simulink model "ITSC2021_CoupledPathFollowingSim_discrete"  (R2019b)
settings: Solver=FixedStepAuto  StartTime=0.0  StopTime=50  FixedStep=0.01  RelTol=1e-4  EnableMultiTasking=on
values from neighbouring files (symbols this model uses):
  friction_grid_cluster = [frictionGrid_Cluster_table.position_x, frictionGrid_Cluster_table.position_y, frictionGrid_Cluster_table.position_z, frictionGrid_Cluster_table.friction_coefficient]    [ITSC2021_runCoupledPathFollowingSim.m]
  inputTrajectory = inputTrajectory(unique_station_indices,:)    [ITSC2021_runCoupledPathFollowingSim.m]
  road_geometry = [sectionRef_table.east, sectionRef_table.north, sectionRef_table.up, sectionRef_table.grade, sectionRef_table.bank, road_geometry_radius, sectionRef_table.yaw]    [ITSC2021_runCoupledPathFollowingSim.m]
undefined symbols (not defined in the file or in its folder): DiscIntNeverNeededParam, flag, initial, mdlparam, mdlParam
libraries: simulink x6, autolibshared x1
(part 1 of 3)
settings Model: Creator=cbeal  LastModifiedBy=LimingGao
settings SolverCC: ZeroCrossAlgorithm=Adaptive
settings DataIOCC: SaveFormat=Array  SaveState=on  SaveTime=off  ReturnWorkspaceOutputs=off
settings OptimizationCC: ExpressionDepthLimit=2147483647  LifeSpan=inf
settings DebuggingCC: ReadBeforeWriteMsg=DisableAll  WriteAfterWriteMsg=DisableAll  WriteAfterReadMsg=DisableAll  UnderspecifiedInitializationDetection=Classic  MergeDetectMultiDrivingBlocksExec=none  SolverPrmCheckMsg=warning  MultiTaskDSMMsg=none  FcnCallInpInsideContextMsg=warning  StateNameClashWarn=warning  SFUnexpectedBacktrackingDiag=warning  SFNoUnconditionalDefaultTransitionDiag=warning  SFExecutionAtInitializationDiag=none  ArithmeticOperatorsInVariantConditions=warning
settings HardwareCC: ProdBitPerPointer=32  ProdBitPerSizeT=32  ProdBitPerPtrDiffT=32  ProdLargestAtomicFloat=None  ProdIntDivRoundTo=Undefined  ProdEndianess=Unspecified  ProdWordSize=32  ProdHWDeviceType=32-bit Generic
settings ModelReferenceCC: UpdateModelReferenceTargets=IfOutOfDate  PropagateSignalLabelsOutOfModel=off
settings SFSimCC: SFSimEcho=off  SimUseLocalCustomCode=off  CustomCodeUndefinedFunction=UseInterfaceOnly
settings RTWCC: RTWUseLocalCustomCode=off
settings CodeAppCC: StateflowObjectComments=on
settings GRTTargetCC: TargetLangStandard=C89/C90 (ANSI)  GeneratePreprocessorConditionals=Disable all
settings ConfigComp: CovMetricSettings=dw  CovHtmlReporting=on  CovSaveCumulativeToWorkspaceVar=on  CovSaveSingleToWorkspaceVar=on  CovExternalEMLEnable=off

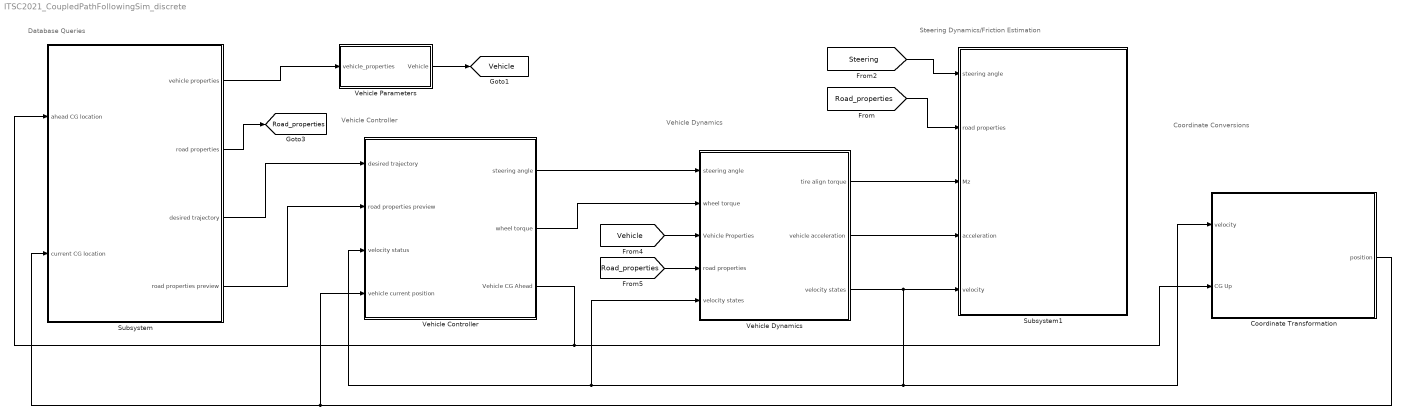
== system ITSC2021_CoupledPathFollowingSim_discrete ==
  note: Steering Dynamics/Friction Estimation
  note: Database Queries
  note: Vehicle Dynamics
  note: Vehicle Controller
  note: Coordinate Conversions
  Coordinate Transformation : Subsystem
  Subsystem : Subsystem
  Subsystem1 : Subsystem
  Vehicle Controller : Subsystem
      mask Display: image('Simulink_MaskIcons\driving_model_icon.png'); % Use "Edit Image" on toolstrip to change.
  Vehicle Dynamics : Subsystem
      mask Display: image('Simulink_MaskIcons\Vehicle_Newton_icon.png'); % Use "Edit Image" on toolstrip to change.
  Vehicle Parameters : Subsystem  mask{vehicleName='C5 Vette', m=1600, m_s=1600, Ixx=0, Iyy=0, Izz=2500, Iw=1.2, Re=0.32, a=1.3, b=1.3, d=1.5, h_cg=0.42, h_rcf=0, h_rcr=0, k_phi=0, b_phi=0, Ca=[95000; 95000; 110000; 110000], Cx=[65000,65000,65000,65000], mu_peak=[1.2 1.2 1.2 1.2], mu_slide=[0.9 0.9 0.9 0.9]}
      mask prompts: vehicleName "Name of Vehicle"; m "Mass"; m_s "Sprung Mass"; Ixx "Roll Moment of Inertia"; Iyy "Pitch Moment of Inertia"; Izz "Yaw Moment of Inertia"; Iw "Wheel Moment of Inertia"; Re "Wheel Effective Radius"; a "CG-Front Axle Distance"; b "CG-Rear Axle Distance"; d "Track Width"; h_cg "CG height"; h_rcf "Front Roll Center Height"; h_rcr "Rear Roll Center Height"; k_phi "Chassis Roll Stiffness (x2)"; b_phi "Chassis Roll Damping (x2)"; Ca "Cornering Stiffnesses (x4)"; Cx "Longitudinal Stiffnesses (x4)"; mu_peak "Peak Coeff. Friction (x4)"; mu_slide "Sliding Coeff. Friction (x4)"
      mask Display: port_label('output',1,vehicleName)
  tag scope: Road_properties=global, Vehicle=global
  wires:
  Vehicle Parameters/1(Vehicle) -> [Vehicle]
  Vehicle Controller/1(steering angle) -> Vehicle Dynamics/1(steering angle)
  Vehicle Controller/3(Vehicle CG Ahead) -> Subsystem/1(ahead CG location), Coordinate Transformation/2(CG Up)
  Vehicle Dynamics/3(" velocity states") -> Coordinate Transformation/1(velocity), Vehicle Dynamics/5(velocity states), Vehicle Controller/3(velocity status), Subsystem1/5(velocity)
  Vehicle Controller/2(wheel torque) -> Vehicle Dynamics/2(wheel torque)
  Subsystem/1(vehicle properties) -> Vehicle Parameters/1(vehicle_properties)
  Subsystem/3(desired trajectory) -> Vehicle Controller/1(desired trajectory)
  Subsystem/4(road properties preview) -> Vehicle Controller/2(road properties preview)
  Coordinate Transformation/1(position) -> Subsystem/2(current CG location), Vehicle Controller/4(vehicle current position)
  Vehicle Dynamics/1(tire align torque) -> Subsystem1/3(Mz)
  Vehicle Dynamics/2(vehicle acceleration) -> Subsystem1/4(acceleration)
  [Steering] -> Subsystem1/1(steering angle)
  [Vehicle] -> Vehicle Dynamics/3(Vehicle Properties)
  Subsystem/2(road properties) -> [Road_properties]
  [Road_properties] -> Vehicle Dynamics/4(road properties)
  [Road_properties] -> Subsystem1/2(road properties)

== system ITSC2021_CoupledPathFollowingSim_discrete/Coordinate Transformation ==
  note: P: Position
      | CG: Center of Gravity
      | ENH: East-North-Heading(yaw angle)
  velocity : Inport
  CG Up : Inport  Port=2
  Body Fixed Coods to World Coords : Subsystem
      mask Display: image('$imagefile'); % Use "Edit Image" on toolstrip to change.
  ENU to LLA : Subsystem
  position : Outport
  wires:
  Body Fixed Coods to World Coords/1(P_CG_ENH) -> ENU to LLA/1(P_CG_ENH1)  "P_CG_ENH"
  ENU to LLA/1(P_CG_ENUH_LLA) -> position/1
  velocity/1 -> Body Fixed Coods to World Coords/1(States)
  CG Up/1 -> ENU to LLA/2(" Up")

== system ITSC2021_CoupledPathFollowingSim_discrete/Subsystem ==
  ahead CG location : Inport
  current CG location : Inport  Port=2
  Bus Creator : BusCreator  Inputs=2
  Bus Creator1 : BusCreator  Inputs=2
  ST Aggregated Prview Friction DB Query : Subsystem
  ST Friction DB Query : Subsystem
  ST Road Geometry DB Query : Subsystem
  ST Trajectory DB Query : Subsystem
  vehicle properties : Outport
  road properties : Outport  Port=2
  desired trajectory : Outport  Port=3
  road properties preview : Outport  Port=4
  wires:
  ST Trajectory DB Query/4(ref_trajectory) -> ST Aggregated Prview Friction DB Query/3(ref_trajectory), ST Road Geometry DB Query/3(ref_trajectory)
  ST Trajectory DB Query/3(trip_status) -> ST Friction DB Query/2(Search_range(segment_id)), ST Road Geometry DB Query/2(Search_range(segment_id)), ST Aggregated Prview Friction DB Query/2(Search_range(segment_id))  "road_segment_id"
  current CG location/1 -> ST Aggregated Prview Friction DB Query/1(Vehicle CG Pose(LLA,ENU,Heading)), ST Road Geometry DB Query/1(Vehicle CG Pose(LLA,ENU,Heading)), ST Friction DB Query/1(Vehicle CG Pose(LLA,ENU,Heading)), ST Trajectory DB Query/2(Vehicle CG Pose(LLA,ENU,Heading))
  ST Trajectory DB Query/2(vehicle_properties) -> vehicle properties/1
  ahead CG location/1 -> ST Trajectory DB Query/1(Vehicle CG Ahead(ENU))
  ST Road Geometry DB Query/2(Road Geometry Preview) -> Bus Creator/1  "Road Geometry Preview"
  ST Trajectory DB Query/1(desired_trajectory) -> desired trajectory/1
  ST Aggregated Prview Friction DB Query/1(Road Friction Preview) -> Bus Creator/2  "Road Friction Preview"
  Bus Creator/1 -> road properties preview/1
  ST Friction DB Query/1(Friction Coefs) -> Bus Creator1/1  "Road Friction"
  Bus Creator1/1 -> road properties/1
  ST Road Geometry DB Query/1(Road Geometry) -> Bus Creator1/2  "Road Geometry"

== system ITSC2021_CoupledPathFollowingSim_discrete/Subsystem1 ==
  steering angle : Inport
  road properties : Inport  Port=2
  Mz : Inport  Port=3
  acceleration : Inport  Port=4
  velocity : Inport  Port=5
  Bus Selector1 : BusSelector  OutputSignals=Road Geometry,Road Friction
  Friction Estimator : Subsystem
  Noise Models : Subsystem
  wires:
  Noise Models/1(Accelerations_est) -> Friction Estimator/4(Accelerations_est)
  acceleration/1 -> Noise Models/2(Accelerations)
  steering angle/1 -> Friction Estimator/6(delta)
  Mz/1 -> Friction Estimator/1(Mz)
  Noise Models/2(States_est) -> Friction Estimator/5(States_est)
  velocity/1 -> Noise Models/1(States)
  road properties/1 -> Bus Selector1/1
  Bus Selector1/1 -> Friction Estimator/2(Road Geometry)  "<Road Geometry>"
  Bus Selector1/2 -> Friction Estimator/3(friction coefficients)  "<Road Friction>"

== system ITSC2021_CoupledPathFollowingSim_discrete/Vehicle Controller ==
  desired trajectory : Inport
  road properties preview : Inport  Port=2
  velocity status : Inport  Port=3
  vehicle current position : Inport  Port=4
  Bus Selector1 : BusSelector  OutputSignals=Road Geometry Preview,Road Friction Preview
  Driver Model : Subsystem
      mask Display: image('$imagefile'); % Use "Edit Image" on toolstrip to change.
  Stabilization : Subsystem
  steering angle : Outport
  wheel torque : Outport  Port=2
  Vehicle CG Ahead : Outport  Port=3
  tag scope: Steering=global
  wires:
  Driver Model/2(Wheel Torques) -> Stabilization/2(torques_driver)
  Stabilization/2(Wheel Torques) -> wheel torque/1
  Driver Model/1(delta) -> Stabilization/1(delta_driver)
  desired trajectory/1 -> Driver Model/2(Desired Trajectory)
  vehicle current position/1 -> Driver Model/3(Vehicle Position)
  Stabilization/1(delta) -> [Steering], steering angle/1
  Driver Model/3(Vehicle CG Ahead) -> Vehicle CG Ahead/1  "current Up = ahead Up"
  velocity status/1 -> Driver Model/1(States)
  Bus Selector1/1 -> Driver Model/4(road_geometry_preview)  "<Road Geometry Preview>"
  road properties preview/1 -> Bus Selector1/1
  Bus Selector1/2 -> Driver Model/5(preview_friction)  "<Road Friction Preview>"

== system ITSC2021_CoupledPathFollowingSim_discrete/Vehicle Dynamics ==
  steering angle : Inport
  wheel torque : Inport  Port=2
  Vehicle Properties : Inport  Port=3
  road properties : Inport  Port=4
  velocity states : Inport  Port=5
  Bus Selector1 : BusSelector  OutputSignals=Road Friction,Road Geometry
  Bus Selector2 : BusSelector  OutputSignals=Road Geometry
  Calculate Normals : Subsystem
  Calculate Slips : Subsystem
  Coupled brush Tire model : Subsystem
      mask Display: image('D:\Box Sync\Research\Project\GitHub\forgetfulDBs\Figures\Simulink_MaskIcons\tire_model_icon2.png'); % Use "Edit Image" on toolstrip to change.
  Vehicle Newtonian Dynamics : Subsystem
      mask Display: image('$imagefile'); % Use "Edit Image" on toolstrip to change.
  road properties1 : InportShadow  Port=4
  tire align torque : Outport
  vehicle acceleration : Outport  Port=2
  " velocity states" : Outport  Port=3
  wires:
  Vehicle Newtonian Dynamics/2(accelerations) -> vehicle acceleration/1, Calculate Normals/2(Accelerations)
  Calculate Normals/1(Normal Forces) -> Coupled brush Tire model/3(normal force)
  steering angle/1 -> Vehicle Newtonian Dynamics/2(delta), Calculate Slips/2(delta)
  Calculate Slips/1(Slips) -> Coupled brush Tire model/1(Slips)
  Bus Selector1/2 -> Calculate Normals/1(Road Geometry)  "<Road Geometry>"
  Coupled brush Tire model/2(Tire Force) -> Vehicle Newtonian Dynamics/4(Tire Forces)
  Vehicle Newtonian Dynamics/1(states) -> " velocity states"/1
  Bus Selector1/1 -> Coupled brush Tire model/2(friction coeffs)  "<Road Friction>"
  velocity states/1 -> Vehicle Newtonian Dynamics/1(States), Calculate Slips/1(States)
  Coupled brush Tire model/1(Align Torque) -> tire align torque/1
  wheel torque/1 -> Vehicle Newtonian Dynamics/3(Wheel Torques)
  Vehicle Properties/1 -> Coupled brush Tire model/4(Vehicle Properties), Vehicle Newtonian Dynamics/6(Vehicle Properties)
  road properties/1 -> Bus Selector1/1
  road properties1/1 -> Bus Selector2/1
  Bus Selector2/1 -> Vehicle Newtonian Dynamics/5(Road Geometry)  "<Road Geometry>"

== system ITSC2021_CoupledPathFollowingSim_discrete/Vehicle Parameters ==
  note: understeer gradient: ku = (mg/l)*(b/Cf - a/Cr)
      | stability factor: k = ku/(lg)=(m/l^2)*(b/Cf - a/Cr) ~10^(-3)
  note: in our model: k = (1600/4.6154)*(0.6/95000-0.4/110000)=0.929*10^-3
      | positive, understeer
  vehicle_properties : Inport
  Add1 : Sum
  Bus Creator : BusCreator  Inputs=19
  Bus Selector1 : BusSelector  OutputSignals=L,d
  Constant : Constant  Value=m
  Constant1 : Constant  Value=Izz
  Constant10 : Constant  Value=Ixx
  Constant11 : Constant  Value=Iyy
  Constant12 : Constant  Value=m_s
  Constant13 : Constant  Value=Re
  Constant14 : Constant  Value=h_cg
  Constant15 : Constant  Value=h_rcf
  Constant16 : Constant  Value=h_rcr
  Constant17 : Constant  Value=k_phi
  Constant18 : Constant  Value=b_phi
  Constant5 : Constant  Value=0.4  VectorParams1D=off  SampleTime=-1
  Constant6 : Constant  Value=0.6  VectorParams1D=off  SampleTime=-1
  Constant7 : Constant  Value=Ca
  Constant8 : Constant  Value=Cx
  Constant9 : Constant  Value=Iw
  Gain : Gain  Gain=1/2
  Product : Product
  Product1 : Product
  Subtract : Sum  Inputs=+-
  Vehicle : Outport
  wires:
  Bus Creator/1 -> Vehicle/1
  Constant/1 -> Bus Creator/1  "m"
  Constant12/1 -> Bus Creator/2  "m_sprung"
  Constant10/1 -> Bus Creator/3  "Ixx"
  Constant11/1 -> Bus Creator/4  "Iyy"
  Constant1/1 -> Bus Creator/5  "Izz"
  Constant9/1 -> Bus Creator/6  "Iw"
  Constant13/1 -> Bus Creator/7  "Re"
  Bus Selector1/1 -> Product/2, Product1/1, Bus Creator/9  "<L>"
  Constant14/1 -> Bus Creator/12, Subtract/1  "h_cg"
  Constant15/1 -> Bus Creator/13, Add1/1  "h_rcf"
  Constant16/1 -> Bus Creator/14, Add1/2  "h_rcr"
  Constant17/1 -> Bus Creator/16  "k_phi"
  Constant18/1 -> Bus Creator/17  "b_phi"
  Constant7/1 -> Bus Creator/18  "Ca"
  Constant8/1 -> Bus Creator/19  "Cx"
  Subtract/1 -> Bus Creator/15  "h1"
  Add1/1 -> Gain/1
  Gain/1 -> Subtract/2
  Product/1 -> Bus Creator/8  "a"
  Bus Selector1/2 -> Bus Creator/11  "<d>"
  Constant6/1 -> Product1/2  "cg rear"
  vehicle_properties/1 -> Bus Selector1/1
  Constant5/1 -> Product/1  "cg front"
  Product1/1 -> Bus Creator/10  "b"

== system ITSC2021_CoupledPathFollowingSim_discrete/Coordinate Transformation/Body Fixed Coods to World Coords ==
  States : Inport
  Bus Creator1 : BusCreator  Inputs=3
  Bus Selector4 : BusSelector  OutputSignals=Vx,Vy,r
  East Discrete-Time Integrator (Forward Euler method one step delay) : DiscreteIntegrator  Commented=on  InitialCondition=initial.east  SampleTime=-1  ICPrevOutput=DiscIntNeverNeededParam  ICPrevScaledInput=DiscIntNeverNeededParam
  East Discrete-Time Integrator (backword Euler method no delay) : DiscreteIntegrator  IntegratorMethod=Integration: Trapezoidal  InitialCondition=initial.east  SampleTime=-1  ICPrevOutput=DiscIntNeverNeededParam  ICPrevScaledInput=DiscIntNeverNeededParam
  East Integrator : Integrator  Commented=on  InitialCondition=initial.east
  North Discrete-Time Integrator : DiscreteIntegrator  Commented=on  InitialCondition=initial.north  SampleTime=-1  ICPrevOutput=DiscIntNeverNeededParam  ICPrevScaledInput=DiscIntNeverNeededParam
  North Discrete-Time Integrator (No delay) : DiscreteIntegrator  IntegratorMethod=Integration: Trapezoidal  InitialCondition=initial.north  SampleTime=-1  ICPrevOutput=DiscIntNeverNeededParam  ICPrevScaledInput=DiscIntNeverNeededParam
  North Integrator : Integrator  Commented=on  InitialCondition=initial.north
  PSI Discrete-Time Integrator : DiscreteIntegrator  Commented=on  InitialCondition=initial.hdg  SampleTime=-1  ICPrevOutput=DiscIntNeverNeededParam  ICPrevScaledInput=DiscIntNeverNeededParam
  PSI Discrete-Time Integrator (backword Euler method no delay) : DiscreteIntegrator  IntegratorMethod=Integration: Trapezoidal  InitialCondition=initial.hdg  SampleTime=-1  ICPrevOutput=DiscIntNeverNeededParam  ICPrevScaledInput=DiscIntNeverNeededParam
  PSI Integrator : Integrator  Commented=on  InitialCondition=initial.hdg
  Product{,1..3} (4 alike) : Product  RndMeth=Zero
  Subtract : Sum
  Subtract1 : Sum  Inputs=-+
  To Workspace1 : ToWorkspace  VariableName=V_east  SampleTime=-1
  To Workspace2 : ToWorkspace  VariableName=Vx  SampleTime=-1
  To Workspace3 : ToWorkspace  VariableName=V_north  SampleTime=-1
  To Workspace4 : ToWorkspace  VariableName=Vy  SampleTime=-1
  To Workspace6 : ToWorkspace  VariableName=P_CG_ENH  SampleTime=-1
  Trigonometric Function : Trigonometry
  Trigonometric Function1 : Trigonometry  Operator=cos
  P_CG_ENH : Outport
  wires:
  PSI Discrete-Time Integrator (backword Euler method no delay)/1 -> Bus Creator1/3, Trigonometric Function/1, Trigonometric Function1/1  "PSI"
  Trigonometric Function/1 -> Product/2, Product1/1
  Product/1 -> Subtract/1
  Trigonometric Function1/1 -> Product2/2, Product3/1
  Product2/1 -> Subtract/2
  Product1/1 -> Subtract1/1
  Product3/1 -> Subtract1/2
  Subtract1/1 -> East Discrete-Time Integrator (backword Euler method no delay)/1, To Workspace1/1
  Subtract/1 -> To Workspace3/1, North Discrete-Time Integrator (No delay)/1
  North Discrete-Time Integrator (No delay)/1 -> Bus Creator1/2  "North"
  East Discrete-Time Integrator (backword Euler method no delay)/1 -> Bus Creator1/1  "East"
  States/1 -> Bus Selector4/1
  Bus Selector4/3 -> PSI Discrete-Time Integrator (backword Euler method no delay)/1  "<r>"
  Bus Selector4/2 -> Product2/1, Product1/2, To Workspace4/1  "<Vy>"
  Bus Selector4/1 -> To Workspace2/1, Product/1, Product3/2  "<Vx>"
  Bus Creator1/1 -> P_CG_ENH/1, To Workspace6/1

== system ITSC2021_CoupledPathFollowingSim_discrete/Coordinate Transformation/ENU to LLA ==
  P_CG_ENH1 : Inport
  " Up" : Inport  Port=2
  Bus Creator : BusCreator  Inputs=7
  Bus Creator2 : BusCreator  Inputs=3
  Bus Selector1 : BusSelector  OutputSignals=East,North
  Bus Selector4 : BusSelector  OutputSignals=East,North,PSI
  Delay to avoid algebraic loop : Delay  Commented=on  DelayLength=1  InitialCondition=0
  Demux1 : Demux  Outputs=3
  IC1 : InitialCondition  Value=0
  P_CG_ENH : InportShadow
  Selector : Selector  InputPortWidth=3  IndexOptions=Index vector (dialog)  Indices=[3]  OutputSizes=1
  To Workspace5 : ToWorkspace  VariableName=P_CG_LLA  SampleTime=-1
  WGS84ENU2LLA : M-S-Function  FunctionName=sfcn_enu2lla  Parameters=mdlparam.refLLA
  P_CG_ENUH_LLA : Outport
  wires:
  Bus Creator2/1 -> WGS84ENU2LLA/1  "ENU"
  WGS84ENU2LLA/1 -> To Workspace5/1, Demux1/1
  P_CG_ENH1/1 -> Bus Selector1/1
  Bus Selector1/1 -> Bus Creator2/1  "<East>"
  Bus Selector1/2 -> Bus Creator2/2  "<North>"
  Selector/1 -> Bus Creator2/3, Bus Creator/4  "UP"
  Demux1/3 -> Bus Creator/7  "Alt"
  Bus Creator/1 -> P_CG_ENUH_LLA/1
  IC1/1 -> Selector/1
  " Up"/1 -> IC1/1
  Demux1/2 -> Bus Creator/6  "Lon"
  Demux1/1 -> Bus Creator/5  "Lat"
  P_CG_ENH/1 -> Bus Selector4/1
  Bus Selector4/2 -> Bus Creator/2  "<North>"
  Bus Selector4/3 -> Bus Creator/3  "<PSI>"
  Bus Selector4/1 -> Bus Creator/1  "<East>"

== system ITSC2021_CoupledPathFollowingSim_discrete/Subsystem/ST Aggregated Prview Friction DB Query ==
  Vehicle CG Pose(LLA,ENU,Heading) : Inport
  Search_range(segment_id) : Inport  Port=2
  ref_trajectory : Inport  Port=3
  Bus Creator1 : BusCreator  Inputs=4
  Bus Creator2 : BusCreator  Inputs=4
  Bus Creator3 : BusCreator  Inputs=2
  Bus Selector : BusSelector  OutputSignals=East,North,UP,PSI
  Bus Selector1 : BusSelector  OutputSignals=Section ID,Total Station,Section Station
  Bus Selector2 : BusSelector  OutputSignals=a,b,d,h_cg
  Constant2 : Constant  Value=friction_grid_cluster
  Terminator : Terminator
  To Workspace1 : ToWorkspace  VariableName=preview_friction  SampleTime=-1
  To Workspace11 : ToWorkspace  VariableName=traj_station  SampleTime=-1
  preview_friction_query : M-S-Function  Commented=on  FunctionName=sfcn_friction_query_preview  Parameters=mdlparam.frictionGridSize,mdlparam.trajectorySize,mdlparam.road_geometry_preview_distance
  Road Friction Preview : Outport
  wires:
  Bus Selector1/1 -> preview_friction_query/4  "<Section ID>"
  Bus Selector/4 -> Bus Creator1/4  "<PSI>"
  Search_range(segment_id)/1 -> Bus Selector1/1
  Bus Selector/2 -> Bus Creator1/2  "<North>"
  Bus Creator1/1 -> preview_friction_query/3  "ENU, yaw"
  Vehicle CG Pose(LLA,ENU,Heading)/1 -> Bus Selector/1
  preview_friction_query/1 -> To Workspace1/1, Road Friction Preview/1
  Bus Selector/1 -> Bus Creator1/1  "<East>"
  Bus Selector2/4 -> Bus Creator2/4  "<h_cg>"
  Constant2/1 -> preview_friction_query/1  "Friction Grid"
  [Vehicle] -> Bus Selector2/1
  Bus Selector/3 -> Bus Creator1/3  "<UP>"
  Bus Selector2/1 -> Bus Creator2/1  "<a>"
  Bus Selector2/2 -> Bus Creator2/2  "<b>"
  Bus Selector2/3 -> Bus Creator2/3  "<d>"
  Bus Selector1/2 -> Bus Creator3/1, preview_friction_query/5  "<Total Station>"
  Bus Selector1/3 -> Bus Creator3/2  "<Section Station>"
  Bus Creator3/1 -> To Workspace11/1
  Bus Creator2/1 -> Terminator/1
  ref_trajectory/1 -> preview_friction_query/2

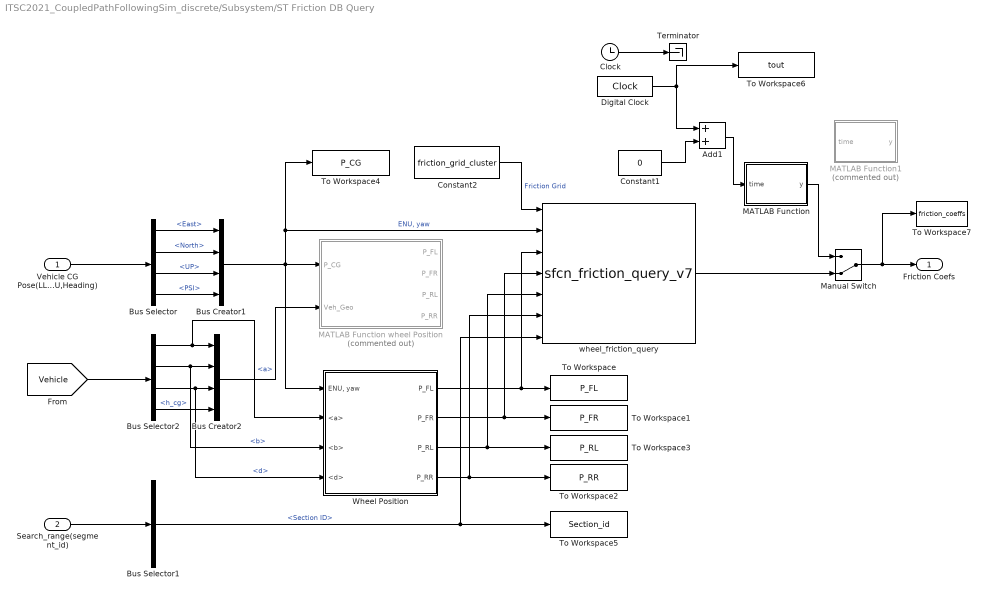
== system ITSC2021_CoupledPathFollowingSim_discrete/Subsystem/ST Friction DB Query ==
  Vehicle CG Pose(LLA,ENU,Heading) : Inport
  Search_range(segment_id) : Inport  Port=2
  Add1 : Sum
  Bus Creator1 : BusCreator  Inputs=4
  Bus Creator2 : BusCreator  Inputs=4
  Bus Selector : BusSelector  OutputSignals=East,North,UP,PSI
  Bus Selector1 : BusSelector  OutputSignals=Section ID
  Bus Selector2 : BusSelector  OutputSignals=a,b,d,h_cg
  Clock : Clock
  Constant1 : Constant  Value=0
  Constant2 : Constant  Value=friction_grid_cluster
  Digital Clock : DigitalClock  SampleTime=0.01
  MATLAB Function : MATLAB Function  TreatAsAtomicUnit=on
      settings: AttributesFormatString=%<SystemSampleTime>
  MATLAB Function wheel Position : MATLAB Function  Commented=on  TreatAsAtomicUnit=on
      settings: AttributesFormatString=|
      | %<SystemSampleTime>
      | %<BlockType>
  MATLAB Function1 : MATLAB Function  Commented=on  TreatAsAtomicUnit=on
  Manual Switch : ManualSwitch  CurrentSetting=0
      settings: AttributesFormatString=%<BlockType>
  Terminator : Terminator
  To Workspace : ToWorkspace  VariableName=P_FL  SampleTime=-1
      settings: Save2DSignal=2-D array (concatenate along first dimension)
  To Workspace1 : ToWorkspace  VariableName=P_FR  SampleTime=-1
      settings: Save2DSignal=2-D array (concatenate along first dimension)
  To Workspace2 : ToWorkspace  VariableName=P_RR  SampleTime=-1
      settings: Save2DSignal=2-D array (concatenate along first dimension)
  To Workspace3 : ToWorkspace  VariableName=P_RL  SampleTime=-1
      settings: Save2DSignal=2-D array (concatenate along first dimension)
  To Workspace4 : ToWorkspace  VariableName=P_CG  SampleTime=-1
      settings: Save2DSignal=2-D array (concatenate along first dimension)
  To Workspace5 : ToWorkspace  VariableName=Section_id  SampleTime=-1
      settings: Save2DSignal=2-D array (concatenate along first dimension)
  To Workspace6 : ToWorkspace  VariableName=tout  SampleTime=-1
      settings: Save2DSignal=2-D array (concatenate along first dimension)
  To Workspace7 : ToWorkspace  VariableName=friction_coeffs  SampleTime=-1
      settings: Save2DSignal=2-D array (concatenate along first dimension)
  Wheel Position : Subsystem
  wheel_friction_query : M-S-Function  FunctionName=sfcn_friction_query_v7  Parameters=mdlparam.frictionGridSize
      settings: AttributesFormatString=BlockType = %<BlockType>
  Friction Coefs : Outport
  wires:
  Bus Creator1/1 -> Wheel Position/1("ENU, yaw"), MATLAB Function wheel Position/1(P_CG), wheel_friction_query/2, To Workspace4/1  "ENU, yaw"
  Bus Creator2/1 -> MATLAB Function wheel Position/2(Veh_Geo)
  Wheel Position/2(P_FR) -> wheel_friction_query/4, To Workspace1/1
  Wheel Position/4(P_RR) -> wheel_friction_query/6, To Workspace2/1
  Wheel Position/1(P_FL) -> wheel_friction_query/3, To Workspace/1
  Wheel Position/3(P_RL) -> wheel_friction_query/5, To Workspace3/1
  Vehicle CG Pose(LLA,ENU,Heading)/1 -> Bus Selector/1
  Constant2/1 -> wheel_friction_query/1  "Friction Grid"
  Bus Selector/1 -> Bus Creator1/1  "<East>"
  Bus Selector/2 -> Bus Creator1/2  "<North>"
  Bus Selector/3 -> Bus Creator1/3  "<UP>"
  Bus Selector/4 -> Bus Creator1/4  "<PSI>"
  wheel_friction_query/1 -> Manual Switch/2
  [Vehicle] -> Bus Selector2/1
  Bus Selector2/1 -> Wheel Position/2(<a>), Bus Creator2/1  "<a>"
  Bus Selector2/2 -> Wheel Position/3(<b>), Bus Creator2/2  "<b>"
  Bus Selector2/3 -> Wheel Position/4(<d>), Bus Creator2/3  "<d>"
  Bus Selector2/4 -> Bus Creator2/4  "<h_cg>"
  Search_range(segment_id)/1 -> Bus Selector1/1
  Bus Selector1/1 -> wheel_friction_query/7, To Workspace5/1  "<Section ID>"
  MATLAB Function/1(y) -> Manual Switch/1
  Manual Switch/1 -> Friction Coefs/1, To Workspace7/1
  Constant1/1 -> Add1/2
  Add1/1 -> MATLAB Function/1(time)
  Clock/1 -> Terminator/1
  Digital Clock/1 -> Add1/1, To Workspace6/1

== system ITSC2021_CoupledPathFollowingSim_discrete/Subsystem/ST Road Geometry DB Query ==
  Vehicle CG Pose(LLA,ENU,Heading) : Inport
  Search_range(segment_id) : Inport  Port=2
  ref_trajectory : Inport  Port=3
  Bus Creator : BusCreator  Inputs=3
  Bus Creator1 : BusCreator  Inputs=4
  Bus Creator2 : BusCreator  Inputs=3
  Bus Selector : BusSelector  OutputSignals=East,North,UP,PSI
  Bus Selector1 : BusSelector  OutputSignals=Section ID
  Constant{1,3..5,19} (5 alike) : Constant  Value=0
  Constant2 : Constant  Value=road_geometry
  To Workspace1 : ToWorkspace  VariableName=preview_radius  SampleTime=-1
  current_road_geometry_query : M-S-Function  Commented=on  FunctionName=sfcn_road_geometry_query  Parameters=mdlparam.frictionGridSize,mdlparam.trajectorySize
  preview_road_geometry_query : M-S-Function  FunctionName=sfcn_road_geometry_query_preview  Parameters=mdlparam.road_geometry,mdlparam.trajectorySize,mdlparam.road_geometry_preview_distance
  Road Geometry : Outport
  Road Geometry Preview : Outport  Port=2
  wires:
  Constant19/1 -> Bus Creator/1  "Bank"
  Bus Creator/1 -> Road Geometry/1
  Constant1/1 -> Bus Creator/2  "Grade"
  Bus Selector/2 -> Bus Creator1/2  "<North>"
  Bus Selector/4 -> Bus Creator1/4  "<PSI>"
  Constant2/1 -> current_road_geometry_query/1, preview_road_geometry_query/1  "road_geometry"
  ref_trajectory/1 -> preview_road_geometry_query/2
  Bus Selector/3 -> Bus Creator1/3  "<UP>"
  Bus Selector/1 -> Bus Creator1/1  "<East>"
  Bus Creator1/1 -> preview_road_geometry_query/3  "ENU, yaw"
  Search_range(segment_id)/1 -> Bus Selector1/1
  Bus Selector1/1 -> preview_road_geometry_query/4  "<Section ID>"
  Vehicle CG Pose(LLA,ENU,Heading)/1 -> Bus Selector/1
  Constant3/1 -> Bus Creator/3  "Curvature"
  Constant5/1 -> Bus Creator2/1  "Bank_preview"
  Constant4/1 -> Bus Creator2/2  "Grade_preview"
  preview_road_geometry_query/1 -> To Workspace1/1, Bus Creator2/3  "Radius_preview"
  Bus Creator2/1 -> Road Geometry Preview/1

== system ITSC2021_CoupledPathFollowingSim_discrete/Subsystem/ST Trajectory DB Query ==
  Vehicle CG Ahead(ENU) : Inport
  Vehicle CG Pose(LLA,ENU,Heading) : Inport  Port=2
  Bus Creator2 : BusCreator  Inputs=3
  Bus Creator3 : BusCreator  Inputs=8
  Bus Creator4 : BusCreator  Inputs=4
  Bus Creator5 : BusCreator  Inputs=8
  Bus Selector : BusSelector  OutputSignals=East,North,UP
  Delay : Delay  Commented=on  DelayLength=1  InitialCondition=0
  Demux : Demux  Outputs=20
  Memory : Memory
  Selector : Selector  NumberOfDimensions=2  InputPortWidth=3  IndexOptions=Starting index (dialog),Starting index (dialog)  Indices=[1],1  OutputSizes=1,20
  To Workspace11 : ToWorkspace  VariableName=Desired_trajectory  SampleTime=-1
  Trajectory Query Block : M-S-Function  FunctionName=sfcn_vehicleTrajectoryFromCurrentAndFuturePos  Parameters=mdlparam.trajectorySize, mdlparam.halfSearchDistance, fieldsPreSimulationVehicleTrajectory, mdlparam.flagFullWndow
      settings: AttributesFormatString=%<BlockType>
  Trajectory Query Block1 : M-S-Function  Commented=on  FunctionName=sfcn_snapPointOntoNearestTrajectory  Parameters=fieldsPreSimulationVehicleTrajectory, mdlparam.halfSearchDistance, mdlparam.trajectorySize
      settings: AttributesFormatString=%<BlockType>
  vehicle_trajectory : Constant  Value=inputTrajectory
  desired_trajectory : Outport
  vehicle_properties : Outport  Port=2
  trip_status : Outport  Port=3
  ref_trajectory : Outport  Port=4
  wires:
  Demux/9 -> Bus Creator3/1  "Des CG Latitude"
  Demux/1 -> Bus Creator4/1  "Vehicle ID"
  Demux/17 -> Bus Creator5/5  "Section Station"
  Demux/8 -> Bus Creator5/4  "Lane Change Flag"
  Trajectory Query Block/1 -> Selector/1
  Selector/1 -> Demux/1
  Demux/13 -> Bus Creator3/5  "Des CG N Coord"
  Demux/20 -> Bus Creator5/8  "Trips ID"
  Demux/10 -> Bus Creator3/2  "Des CG Longitude"
  Demux/11 -> Bus Creator3/3  "Des CG Altitude"
  Bus Creator5/1 -> trip_status/1
  Bus Creator3/1 -> To Workspace11/1, desired_trajectory/1
  Vehicle CG Ahead(ENU)/1 -> Trajectory Query Block/3
  Demux/15 -> Bus Creator3/7  "Des Hdg Angle"
  Demux/18 -> Bus Creator5/6  "Total Station"
  Demux/7 -> Bus Creator5/3  "Lane Number"
  vehicle_trajectory/1 -> ref_trajectory/1, Trajectory Query Block/1
  Bus Creator4/1 -> vehicle_properties/1
  Demux/4 -> Bus Creator4/4  "d"
  Demux/12 -> Bus Creator3/4  "Des CG E Coord"
  Demux/19 -> Bus Creator5/7  "AIMSUN Time"
  Demux/14 -> Memory/1  "Des CG U Coord"
  Demux/5 -> Bus Creator5/1  "Section ID"
  Demux/6 -> Bus Creator5/2  "Junction ID"
  Demux/16 -> Bus Creator3/8  "Des Path Speed"
  Demux/3 -> Bus Creator4/3  "L"
  Demux/2 -> Bus Creator4/2  "Vehicle Type"
  Bus Selector/3 -> Bus Creator2/3  "<UP>"
  Vehicle CG Pose(LLA,ENU,Heading)/1 -> Bus Selector/1
  Bus Selector/1 -> Bus Creator2/1  "<East>"
  Bus Selector/2 -> Bus Creator2/2  "<North>"
  Bus Creator2/1 -> Trajectory Query Block/2  "ENU"
  Memory/1 -> Bus Creator3/6  "Des CG U Coord"

== system ITSC2021_CoupledPathFollowingSim_discrete/Subsystem1/Friction Estimator ==
  Mz : Inport
  Road Geometry : Inport  Port=2
  friction coefficients : Inport  Port=3
  Accelerations_est : Inport  Port=4
  States_est : Inport  Port=5
  delta : Inport  Port=6
  Friction Coefficients Estimate : Subsystem
  To Workspace1 : ToWorkspace  VariableName=friction_coeffs_estimate  SampleTime=-1
  fric est Calculate Normals : Subsystem
  fric est Calculate Slips : Subsystem
  fric est Calculate Xis : Subsystem
  wires:
  States_est/1 -> fric est Calculate Slips/1(States_est)
  delta/1 -> fric est Calculate Slips/2(delta)
  Accelerations_est/1 -> fric est Calculate Normals/2(Accelerations)
  Road Geometry/1 -> fric est Calculate Normals/1(Road Geometry)
  fric est Calculate Slips/1(Slip Angles est) -> fric est Calculate Xis/2(Slip Angles est)
  Friction Coefficients Estimate/1(friction coefficients Estimate) -> To Workspace1/1
  fric est Calculate Xis/1(fric est coefficients) -> Friction Coefficients Estimate/2(fric est coefficients)
  Mz/1 -> Friction Coefficients Estimate/1(Mz)
  fric est Calculate Normals/1(Normal Forces) -> Friction Coefficients Estimate/3(fric est Normal Forces)
  friction coefficients/1 -> fric est Calculate Xis/1(friction coefficients)

== system ITSC2021_CoupledPathFollowingSim_discrete/Subsystem1/Noise Models ==
  States : Inport
  Accelerations : Inport  Port=2
  Bus Creator1 : BusCreator  Inputs=3
  Bus Creator2 : BusCreator  Inputs=2
  Bus Selector2 : BusSelector  OutputSignals=Vx,Vy,r
  Bus Selector3 : BusSelector  OutputSignals=ax,ay
  GPS Noise Function : MATLAB Function  TreatAsAtomicUnit=on
  IMU Noise Function : MATLAB Function  TreatAsAtomicUnit=on
  Sampling Time : Constant  Value=mdlParam.sampling_time
  Sampling Time1 : Constant  Value=mdlParam.sampling_time_accel
  To Workspace1 : ToWorkspace  VariableName=ax_est  SampleTime=-1
  To Workspace2 : ToWorkspace  VariableName=Vx_est  SampleTime=-1
  To Workspace3 : ToWorkspace  VariableName=Vy_est  SampleTime=-1
  To Workspace4 : ToWorkspace  VariableName=ay_est  SampleTime=-1
  To Workspace5 : ToWorkspace  VariableName=r_est  SampleTime=-1
  Accelerations_est : Outport
  States_est : Outport  Port=2
  wires:
  Bus Selector2/3 -> GPS Noise Function/3(r)  "<r>"
  States/1 -> Bus Selector2/1
  Bus Selector2/2 -> GPS Noise Function/2(v_y)  "<Vy>"
  Bus Selector2/1 -> GPS Noise Function/1(v_x)  "<Vx>"
  Bus Creator1/1 -> States_est/1
  Bus Selector3/1 -> IMU Noise Function/1(a_x)  "<ax>"
  Bus Selector3/2 -> IMU Noise Function/2(a_y)  "<ay>"
  Accelerations/1 -> Bus Selector3/1
  GPS Noise Function/3(r_out) -> To Workspace5/1, Bus Creator1/3
  Bus Creator2/1 -> Accelerations_est/1
  Sampling Time/1 -> GPS Noise Function/4(sampling_time)
  GPS Noise Function/1(v_x_out) -> To Workspace2/1, Bus Creator1/1
  GPS Noise Function/2(v_y_out) -> To Workspace3/1, Bus Creator1/2
  IMU Noise Function/2(a_y_out) -> To Workspace4/1, Bus Creator2/2
  IMU Noise Function/1(a_x_out) -> To Workspace1/1, Bus Creator2/1
  Sampling Time1/1 -> IMU Noise Function/3(sampling_time)

== system ITSC2021_CoupledPathFollowingSim_discrete/Vehicle Controller/Driver Model ==
  States : Inport
  Desired Trajectory : Inport  Port=2
  Vehicle Position : Inport  Port=3
  road_geometry_preview : Inport  Port=4
  preview_friction : Inport  Port=5
  Drive Line : Subsystem
  Longitudinal Driver : autolibshared/Longitudinal Driver  Commented=on  cntrlType=PI  shftType=None  velUnits=m/s  gearOut=off  Kp=10  Ki=5  Kff=.1  Kg=0  VehVelVec=[0 100]  KffVec=[.1 .1]  KpVec=[10 10]  KiVec=[5 5]  KgVec=[0 0]  m=1500  Kpt=3000  tau=.1  L=2  aR=200  bR=2.5  cR=.5  g=9.81  vnom=5  Kaw=1  tauerr=.01  tauPt=2  GearInit=0  tShift=.1  pdlVec=[0.1 0.4 0.5 0.9]  upShftTbl=[-1 12.9375 26.4375 39.9375 51.18749999999999 62.4375 72.84375 83.25;-1 16.3125 29.8125 43.3125 54.5624 65.8125 76.78125 87.75;-1 19.6875 33.1875 46.68749999999999 57.9375 69.1875 80.71875 92.25;-1 33 52.5 77.25 100.5 138.75 161.875 185]  dwnShftTbl=[1 9.5625 23.0625 36.5625 47.8125 59.0625 68.90625 78.75;1 12.9375 26.4375 39.9375 51.18749999999999 62.4375 72.84375 83.25;1 16.3125 29.8125 43.3125 54.562499 65.8125 76.78125 87.75;1 19.6875 33.1875 46.68749999999999 57.9375 69.1875 80.71875 92.25]  tClutch=.5  tRev=.5  tPark=120  aMode=2  UpGearVec="[0  1  2  3  4  5  6  7]"  DownGearVec="[1  2  3  4  5  6  7  8]"
      settings: SourceProductName=Powertrain Blockset  SourceProductBaseCode=PW
  Steering : Subsystem
  delta : Outport
  Wheel Torques : Outport  Port=2
  Vehicle CG Ahead : Outport  Port=3
  wires:
  Desired Trajectory/1 -> Steering/1(Desired Trajectory), Drive Line/4(Desired Trajectory)
  Vehicle Position/1 -> Steering/2(Vehicle Position)
  Steering/1(steering angle) -> delta/1
  Steering/2(Vehicle CG Ahead) -> Vehicle CG Ahead/1
  States/1 -> Drive Line/1(States)
  road_geometry_preview/1 -> Drive Line/2(road_geometry_preview)
  preview_friction/1 -> Drive Line/3(preview_friction)
  Drive Line/1(Wheel Torques) -> Wheel Torques/1

== system ITSC2021_CoupledPathFollowingSim_discrete/Vehicle Controller/Stabilization ==
  delta_driver : Inport
  torques_driver : Inport  Port=2
  Gain : Gain
  Gain1 : Gain
  To Workspace12 : ToWorkspace  VariableName=wheel_torques  SampleTime=-1
  To Workspace3 : ToWorkspace  VariableName=delta  SampleTime=-1
  steering angle limitation : Saturate  UpperLimit=30*pi/180  LowerLimit=-30*pi/180
  torque limitation : Saturate  UpperLimit=200  LowerLimit=-400
  delta : Outport
  Wheel Torques : Outport  Port=2
  wires:
  torques_driver/1 -> Gain/1
  delta_driver/1 -> Gain1/1
  Gain/1 -> torque limitation/1
  Gain1/1 -> steering angle limitation/1
  torque limitation/1 -> To Workspace12/1, Wheel Torques/1
  steering angle limitation/1 -> To Workspace3/1, delta/1

== system ITSC2021_CoupledPathFollowingSim_discrete/Vehicle Dynamics/Calculate Normals ==
  Road Geometry : Inport
  Accelerations : Inport  Port=2
  Left Front : Sum  Inputs=+--
  Left Rear : Sum  Inputs=++-
  Mux : Mux
  Normal Force Lateral Transfer : Subsystem
  Normal Force Longitudinal Transfer : Subsystem
  Normal Force Static : Subsystem
  Right Front : Sum  Inputs=+-+
  Right Rear : Sum  Inputs=+++
  To Workspace6 : ToWorkspace  VariableName=Fz  SampleTime=-1
  Normal Forces : Outport
  wires:
  Mux/1 -> Normal Forces/1, To Workspace6/1
  Left Front/1 -> Mux/1
  Right Front/1 -> Mux/2
  Left Rear/1 -> Mux/3
  Right Rear/1 -> Mux/4
  Normal Force Static/2(Half Static Rear) -> Right Rear/1, Left Rear/1
  Normal Force Static/1(Half Static Front) -> Left Front/1, Right Front/1
  Road Geometry/1 -> Normal Force Static/1(Road Geometry)
  Normal Force Longitudinal Transfer/1(Half Long Transfer) -> Left Front/2, Right Front/2, Left Rear/2, Right Rear/2
  Accelerations/1 -> Normal Force Lateral Transfer/1(Accelerations), Normal Force Longitudinal Transfer/1(Accelerations)
  Normal Force Lateral Transfer/2(Lateral Transfer Rear) -> Left Rear/3, Right Rear/3
  Normal Force Lateral Transfer/1(Lateral Transfer Front) -> Left Front/3, Right Front/3

== system ITSC2021_CoupledPathFollowingSim_discrete/Vehicle Dynamics/Calculate Slips ==
  States : Inport
  delta : Inport  Port=2
  Bus Creator1 : BusCreator  Inputs=2
  Slip Angle : Subsystem
  Terminator2 : Terminator
  To Workspace : ToWorkspace  VariableName=alpha  SampleTime=-1
  To Workspace1 : ToWorkspace  Commented=on  VariableName=kappa1  SampleTime=-1
  To Workspace2 : ToWorkspace  VariableName=kappa  SampleTime=-1
  Wheel Slip Ratio this block is wrong because it use vehicle body velocity to calculate slip ratio : Subsystem  Commented=on
  Wheel Slip Ratio1 : Subsystem
  vehicle2tire : Subsystem
  Slips : Outport
  wires:
  Bus Creator1/1 -> Slips/1
  Slip Angle/1(Slip Angles) -> Bus Creator1/1, To Workspace/1  "Slip Angles"
  Wheel Slip Ratio this block is wrong because it use vehicle body velocity to calculate slip ratio/1(Wheel Slips) -> To Workspace1/1  "Wheel Slip Ratio"
  States/1 -> Wheel Slip Ratio this block is wrong because it use vehicle body velocity to calculate slip ratio/1(States), Wheel Slip Ratio1/2(States), vehicle2tire/1(States), Slip Angle/2(States)  "vx,vy,r,omega"
  delta/1 -> vehicle2tire/2(delta), Slip Angle/1(delta)
  vehicle2tire/2(Vtire,y) -> Terminator2/1
  vehicle2tire/1(Vtire,x) -> Wheel Slip Ratio1/1(Vtire,x)
  Wheel Slip Ratio1/1(Wheel Slips Ratio) -> Bus Creator1/2, To Workspace2/1  "Wheel Slip Ratio"

== system ITSC2021_CoupledPathFollowingSim_discrete/Vehicle Dynamics/Coupled brush Tire model ==
  note: [1] J. Svendenius, “Tire Modeling and Friction Estimation,” Control , p. 194, 2007. chapter2.4 and chapter4
      | [2] M. Kissai et al. , “A new linear tire model with varying parameters To cite this version : HAL Id : hal-01690792 A New Linear Tire Model With Varying Parameters,” 2018.
  Slips : Inport
  friction coeffs : Inport  Port=2
  normal force : Inport  Port=3
  Vehicle Properties : Inport  Port=4
  Brush Aligning Moment Model : Subsystem
  Constant3 : Constant
  Switch1 : Switch  Threshold=1  ZeroCross=off
  Wheel Forces : Subsystem
  tire slip : Subsystem
  Align Torque : Outport
  Tire Force : Outport  Port=2
  wires:
  Switch1/1 -> Wheel Forces/6(Psi_Tire)
  normal force/1 -> Brush Aligning Moment Model/2(Normal Forces), Wheel Forces/2(normal force), tire slip/3(normal force)
  Wheel Forces/1(Forces) -> Tire Force/1
  tire slip/4(Psi_Tire) -> Switch1/3, Switch1/2
  tire slip/1(sigma_x) -> Wheel Forces/3(sigma_x)
  friction coeffs/1 -> Brush Aligning Moment Model/3(Friction Coefficients), Wheel Forces/1(sliding friction), tire slip/2(peak friction)  "assume: sliding friction coefficient = adhesive friction coefficient"
  Slips/1 -> Brush Aligning Moment Model/1(Slips), tire slip/1(Slips)
  tire slip/2(sigma_y) -> Wheel Forces/4(sigma_y)
  tire slip/3(sigma) -> Wheel Forces/5(sigma)
  Constant3/1 -> Switch1/1  "Pure Sliding"
  Brush Aligning Moment Model/1(Mz) -> Align Torque/1
  Vehicle Properties/1 -> tire slip/4(Vehicle Properties)

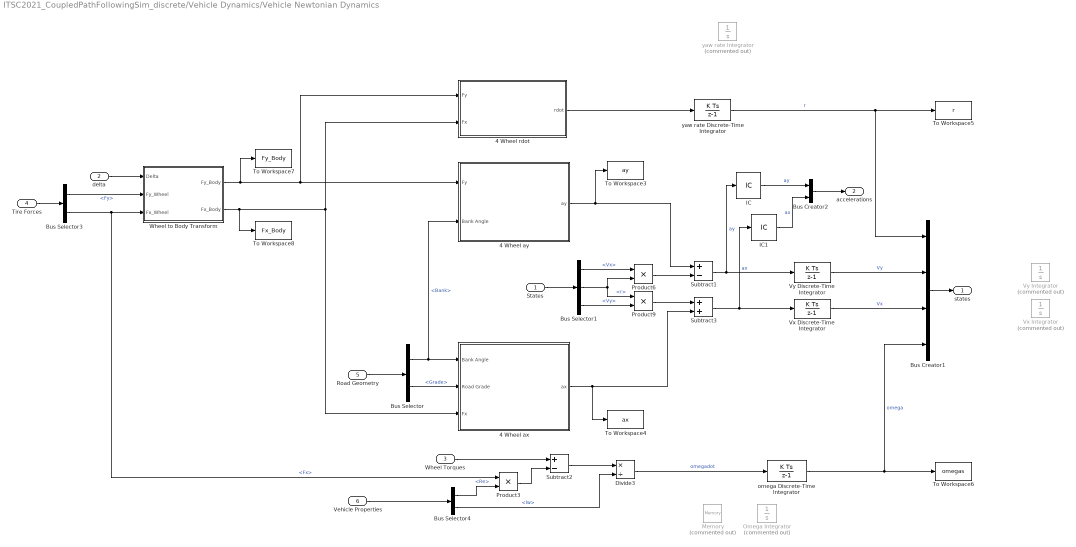
== system ITSC2021_CoupledPathFollowingSim_discrete/Vehicle Dynamics/Vehicle Newtonian Dynamics ==
  States : Inport
  delta : Inport  Port=2
  Wheel Torques : Inport  Port=3
  Tire Forces : Inport  Port=4
  Road Geometry : Inport  Port=5
  Vehicle Properties : Inport  Port=6
  4 Wheel ax : Subsystem
  4 Wheel ay : Subsystem
  4 Wheel rdot : Subsystem
  Bus Creator1 : BusCreator  Inputs=4
  Bus Creator2 : BusCreator  Inputs=2
  Bus Selector : BusSelector  OutputSignals=Bank,Grade
  Bus Selector1 : BusSelector  OutputSignals=Vx,r,Vy
  Bus Selector3 : BusSelector  OutputSignals=Fy,Fx
  Bus Selector4 : BusSelector  OutputSignals=Re,Iw
  Divide3 : Product  Inputs=*/
  IC : InitialCondition  Value=0
  IC1 : InitialCondition  Value=0
  Memory : Memory  Commented=on  InitialCondition=initial.wheelspeeds  InheritSampleTime=on
  Omega Integrator : Integrator  Commented=on  InitialCondition=initial.wheelspeeds
  Product3 : Product  RndMeth=Zero
  Product6 : Product  RndMeth=Zero
  Product9 : Product  RndMeth=Zero
  Subtract1 : Sum  Inputs=+-
  Subtract2 : Sum  Inputs=+-
  Subtract3 : Sum
  To Workspace3 : ToWorkspace  VariableName=ay  SampleTime=-1
  To Workspace4 : ToWorkspace  VariableName=ax  SampleTime=-1
  To Workspace5 : ToWorkspace  VariableName=r  SampleTime=-1
  To Workspace6 : ToWorkspace  VariableName=omegas  SampleTime=-1
  To Workspace7 : ToWorkspace  VariableName=Fy_Body  SampleTime=-1
  To Workspace8 : ToWorkspace  VariableName=Fx_Body  SampleTime=-1
  Vx Discrete-Time Integrator : DiscreteIntegrator  InitialCondition=initial.speed  SampleTime=-1  ICPrevOutput=DiscIntNeverNeededParam  ICPrevScaledInput=DiscIntNeverNeededParam
  Vx Integrator : Integrator  Commented=on  InitialCondition=initial.speed
  Vy Discrete-Time Integrator : DiscreteIntegrator  gainval=1  SampleTime=-1  ICPrevOutput=DiscIntNeverNeededParam  ICPrevScaledInput=DiscIntNeverNeededParam
  Vy Integrator : Integrator  Commented=on  InitialCondition=0.0001
  Wheel to Body Transform : Subsystem
  omega Discrete-Time Integrator : DiscreteIntegrator  InitialCondition=initial.wheelspeeds  SampleTime=-1  ICPrevOutput=DiscIntNeverNeededParam  ICPrevScaledInput=DiscIntNeverNeededParam
  yaw rate Discrete-Time Integrator : DiscreteIntegrator  SampleTime=-1  ICPrevOutput=DiscIntNeverNeededParam  ICPrevScaledInput=DiscIntNeverNeededParam
  yaw rate Integrator : Integrator  Commented=on
  states : Outport
  accelerations : Outport  Port=2
  wires:
  Vehicle Properties/1 -> Bus Selector4/1
  Bus Selector4/2 -> Divide3/2  "<Iw>"
  Bus Selector4/1 -> Product3/2  "<Re>"
  Product3/1 -> Subtract2/2
  Wheel Torques/1 -> Subtract2/1
  Subtract2/1 -> Divide3/1
  Divide3/1 -> omega Discrete-Time Integrator/1  "omegadot"
  yaw rate Discrete-Time Integrator/1 -> To Workspace5/1, Bus Creator1/1  "r"
  Vy Discrete-Time Integrator/1 -> Bus Creator1/2  "Vy"
  Vx Discrete-Time Integrator/1 -> Bus Creator1/3  "Vx"
  omega Discrete-Time Integrator/1 -> To Workspace6/1, Bus Creator1/4  "omega"
  IC/1 -> Bus Creator2/1  "ay"
  IC1/1 -> Bus Creator2/2  "ax"
  Bus Creator2/1 -> accelerations/1
  Product6/1 -> Subtract1/2
  Subtract1/1 -> Vy Discrete-Time Integrator/1, IC/1  "ay"
  Product9/1 -> Subtract3/1
  Subtract3/1 -> IC1/1, Vx Discrete-Time Integrator/1  "ax"
  Bus Selector/2 -> 4 Wheel ax/2(Road Grade)  "<Grade>"
  Wheel to Body Transform/1(Fy_Body) -> 4 Wheel ay/1(Fy), 4 Wheel rdot/1(Fy), To Workspace7/1
  Wheel to Body Transform/2(Fx_Body) -> 4 Wheel ax/3("Fx "), 4 Wheel rdot/2(Fx), To Workspace8/1
  4 Wheel rdot/1(rdot) -> yaw rate Discrete-Time Integrator/1
  4 Wheel ay/1(ay) -> To Workspace3/1, Subtract1/1
  4 Wheel ax/1(ax) -> To Workspace4/1, Subtract3/2
  Bus Creator1/1 -> states/1
  Bus Selector/1 -> 4 Wheel ax/1(Bank Angle), 4 Wheel ay/2(Bank Angle)  "<Bank>"
  Road Geometry/1 -> Bus Selector/1
  delta/1 -> Wheel to Body Transform/1(Delta)
  States/1 -> Bus Selector1/1
  Bus Selector1/1 -> Product6/1  "<Vx>"
  Bus Selector1/3 -> Product9/2  "<Vy>"
  Bus Selector1/2 -> Product9/1, Product6/2  "<r>"
  Tire Forces/1 -> Bus Selector3/1
  Bus Selector3/2 -> Product3/1, Wheel to Body Transform/3(Fx_Wheel)  "<Fx>"
  Bus Selector3/1 -> Wheel to Body Transform/2(Fy_Wheel)  "<Fy>"

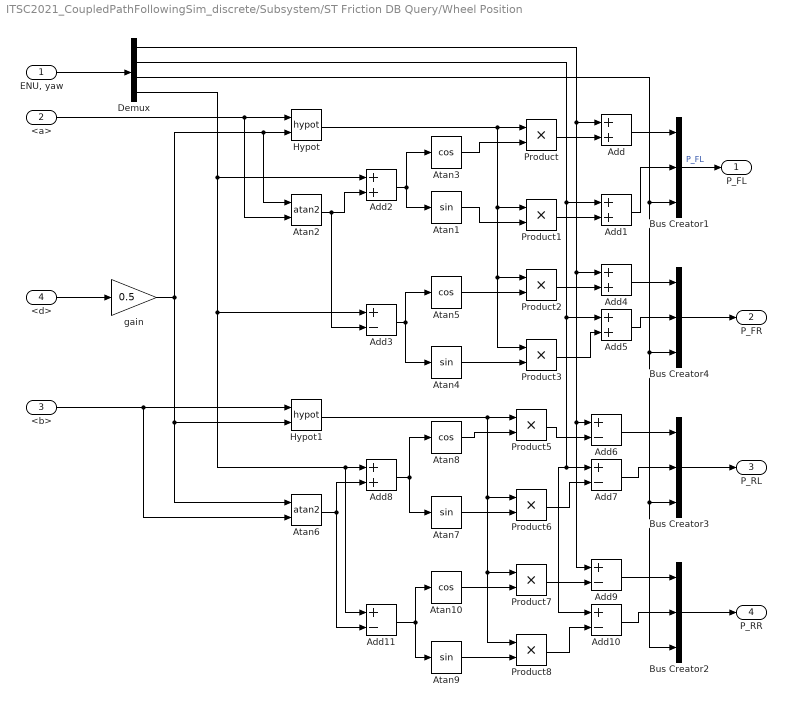
== system ITSC2021_CoupledPathFollowingSim_discrete/Subsystem/ST Friction DB Query/Wheel Position ==
  "ENU, yaw" : Inport
  <a> : Inport  Port=2
  <b> : Inport  Port=3
  <d> : Inport  Port=4
  Add{,1..2,4..5,8} (6 alike) : Sum
  Add{3,6..7,9..11} (6 alike) : Sum  Inputs=+-
  Atan{1,4,7,9} (4 alike) : Trigonometry
  Atan{3,5,8,10} (4 alike) : Trigonometry  Operator=cos
  Atan2 : Trigonometry  Operator=atan2
  Atan6 : Trigonometry  Operator=atan2
  Bus Creator{1..4} (4 alike) : BusCreator  Inputs=3
  Demux : Demux
  Hypot : Math  Operator=hypot  SignedPower=off  SaturateOnIntegerOverflow=on
  Hypot1 : Math  Operator=hypot  SignedPower=off  SaturateOnIntegerOverflow=on
  Product{,1..3,5..8} (8 alike) : Product
  gain : Gain  Gain=0.5  SaturateOnIntegerOverflow=on  OutDataTypeStr=Inherit: Same as input  ParamDataTypeStr=Inherit: Same as input
  P_FL : Outport
  P_FR : Outport  Port=2
  P_RL : Outport  Port=3
  P_RR : Outport  Port=4
  wires:
  Add10/1 -> Bus Creator2/2
  Demux/4 -> Add2/1, Add11/1, Add8/1, Add3/1
  Atan1/1 -> Product1/2
  Hypot/1 -> Product2/1, Product3/1, Product1/1, Product/1
  Demux/1 -> Add9/1, Add6/1, Add4/1, Add/1
  <b>/1 -> Atan6/2, Hypot1/1
  <d>/1 -> gain/1
  Product3/1 -> Add5/2
  Atan2/1 -> Add3/2, Add2/2
  Bus Creator2/1 -> P_RR/1
  Demux/3 -> Bus Creator2/3, Bus Creator3/3, Bus Creator4/3, Bus Creator1/3
  gain/1 -> Atan6/1, Hypot1/2, Atan2/1, Hypot/2
  Product1/1 -> Add1/2
  Hypot1/1 -> Product7/1, Product8/1, Product6/1, Product5/1
  Demux/2 -> Add5/1, Add10/1, Add7/1, Add1/1
  Product8/1 -> Add10/2
  Product/1 -> Add/2
  <a>/1 -> Atan2/2, Hypot/1
  Product5/1 -> Add6/2
  Bus Creator4/1 -> P_FR/1
  Atan7/1 -> Product6/2
  Bus Creator3/1 -> P_RL/1
  Add3/1 -> Atan5/1, Atan4/1
  Product6/1 -> Add7/2
  Atan8/1 -> Product5/2
  Add9/1 -> Bus Creator2/1
  Atan9/1 -> Product8/2
  Add4/1 -> Bus Creator4/1
  Add2/1 -> Atan1/1, Atan3/1
  Atan3/1 -> Product/2
  Add/1 -> Bus Creator1/1
  Add7/1 -> Bus Creator3/2
  Atan6/1 -> Add11/2, Add8/2
  Atan4/1 -> Product3/2
  Atan5/1 -> Product2/2
  Add8/1 -> Atan7/1, Atan8/1
  Add5/1 -> Bus Creator4/2
  Product2/1 -> Add4/2
  Product7/1 -> Add9/2
  Add1/1 -> Bus Creator1/2
  Atan10/1 -> Product7/2
  Add11/1 -> Atan9/1, Atan10/1
  Add6/1 -> Bus Creator3/1
  Bus Creator1/1 -> P_FL/1  "P_FL"
  "ENU, yaw"/1 -> Demux/1

== system ITSC2021_CoupledPathFollowingSim_discrete/Subsystem1/Friction Estimator/Friction Coefficients Estimate ==
  Mz : Inport
  fric est coefficients : Inport  Port=2
  fric est Normal Forces : Inport  Port=3
  Demux1 : Demux
  Divide : Product  Inputs=*/
  Estimate Friction Force : M-S-Function  FunctionName=sfcn_estimateFrictionForce
  To Workspace5 : ToWorkspace  VariableName=frictionalForce_est  SampleTime=-1
  friction coefficients Estimate : Outport
  wires:
  fric est coefficients/1 -> Demux1/1
  Estimate Friction Force/1 -> Divide/1, To Workspace5/1
  Mz/1 -> Estimate Friction Force/1
  Demux1/1 -> Estimate Friction Force/2  "Xi1"
  Demux1/2 -> Estimate Friction Force/3  "Xi2"
  Demux1/3 -> Estimate Friction Force/4  "Xi3"
  Demux1/4 -> Estimate Friction Force/5  "Xi4"
  fric est Normal Forces/1 -> Divide/2
  Divide/1 -> friction coefficients Estimate/1

== system ITSC2021_CoupledPathFollowingSim_discrete/Subsystem1/Friction Estimator/fric est Calculate Normals ==
  Road Geometry : Inport
  Accelerations : Inport  Port=2
  Left Front : Sum  Inputs=+--
  Left Rear : Sum  Inputs=++-
  Mux : Mux
  Normal Force Lateral Transfer : Subsystem
  Normal Force Longitudinal Transfer : Subsystem
  Normal Force Static : Subsystem
  Right Front : Sum  Inputs=+-+
  Right Rear : Sum  Inputs=+++
  Normal Forces : Outport
  wires:
  Mux/1 -> Normal Forces/1
  Left Front/1 -> Mux/1
  Right Front/1 -> Mux/2
  Left Rear/1 -> Mux/3
  Right Rear/1 -> Mux/4
  Normal Force Static/2(Half Static Rear) -> Right Rear/1, Left Rear/1
  Normal Force Static/1(Half Static Front) -> Left Front/1, Right Front/1
  Road Geometry/1 -> Normal Force Static/1(Road Geometry)
  Normal Force Longitudinal Transfer/1(Half Long Transfer) -> Left Front/2, Right Front/2, Left Rear/2, Right Rear/2
  Accelerations/1 -> Normal Force Lateral Transfer/1(Accelerations), Normal Force Longitudinal Transfer/1(Accelerations)
  Normal Force Lateral Transfer/2(Lateral Transfer Rear) -> Left Rear/3, Right Rear/3
  Normal Force Lateral Transfer/1(Lateral Transfer Front) -> Left Front/3, Right Front/3
